simulink model "KugleSim_SlidingMode"  (R2018a)
settings: Solver=VariableStepAuto  StartTime=0.0  StopTime=5  FixedStep=1e-3  MaxStep=1e-2  RelTol=1e-5
PreLoadFcn:
  | modelDir = fileparts(get_param(bdroot, 'FileName'));
  | addpath(fullfile(modelDir,'../Parameters'));
  | addpath(fullfile(modelDir,'subsystems'));
  | 
  | Parameters_General
  | Parameters_Simulation
  | Parameters_Controllers
InitFcn:
  | Parameters_General
  | Parameters_Simulation
  | Parameters_Controllers
StopFcn:
  | StructurizeLoggedData
values from neighbouring files (symbols this model uses):
  Ts = 1/200    (= 0.005)    [Parameters_Controller.m]
settings Model: Creator=Thomas  LastModifiedBy=Thomas
settings DebuggingCC: UniqueDataStoreMsg=error
settings HardwareCC: ProdBitPerPointer=32  ProdBitPerSizeT=32  ProdBitPerPtrDiffT=32  ProdLargestAtomicInteger=Long  ProdLargestAtomicFloat=Double  ProdWordSize=32  ProdHWDeviceType=ARM Compatible->ARM Cortex
settings ModelReferenceCC: ModelReferenceNumInstancesAllowed=Zero
settings RTWCC: GenCodeOnly=on  Toolchain=GNU Tools for ARM Embedded Processors
settings GRTTargetCC: TargetLangStandard=C89/C90 (ANSI)  CodeReplacementLibrary=ARM Cortex-M (CMSIS)

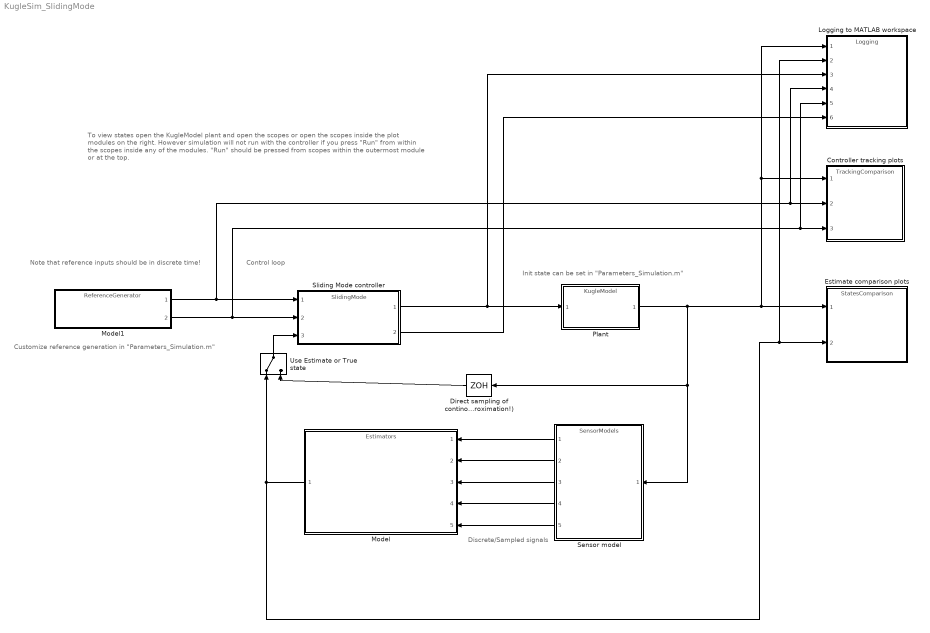
== system KugleSim_SlidingMode ==
  note: Control loop
  note: Discrete/Sampled signals
  note: Init state can be set in "Parameters_Simulation.m"
  note: To view states open the KugleModel plant and open the scopes or open the scopes inside the plot modules on the right.
      | However simulation will not run with the controller if you press "Run" from within the scopes inside any of the modules.
      | "Run" should be pressed from scopes within the outermost module or at the top.
  note: Note that reference inputs should be in discrete time!
  note: Customize reference generation in "Parameters_Simulation.m"
  Controller tracking plots : ModelReference  ModelNameDialog=TrackingComparison  SimulationMode=Normal  ModelReferenceVersion=1.12
  Direct sampling of continous states (simple/approximation!) : ZeroOrderHold  SampleTime=Ts
  Estimate comparison plots : ModelReference  ModelNameDialog=StatesComparison  SimulationMode=Normal  ModelReferenceVersion=1.9
  Logging to MATLAB workspace : ModelReference  ModelNameDialog=Logging  SimulationMode=Normal  ModelReferenceVersion=1.12
  Model : ModelReference  ModelNameDialog=Estimators  SimulationMode=Normal  ModelReferenceVersion=1.10
  Model1 : ModelReference  ModelNameDialog=ReferenceGenerator  SimulationMode=Normal  ModelReferenceVersion=1.7
  Plant : ModelReference  ModelNameDialog=KugleModel  SimulationMode=Normal  ModelReferenceVersion=1.2090
  Sensor model : ModelReference  ModelNameDialog=SensorModels  SimulationMode=Normal  ModelReferenceVersion=1.18
  Sliding Mode controller : ModelReference  ModelNameDialog=SlidingMode  SimulationMode=Normal  ModelReferenceVersion=1.48
  Use Estimate or True state : ManualSwitch
  wires:
  Direct sampling of continous states (simple/approximation!)/1 -> Use Estimate or True state/2
  Plant/1 -> Sensor model/1, Direct sampling of continous states (simple/approximation!)/1, Logging to MATLAB workspace/1, Controller tracking plots/1, Estimate comparison plots/1
  Model1/2 -> Logging to MATLAB workspace/5, Controller tracking plots/3, Sliding Mode controller/2
  Sliding Mode controller/1 -> Logging to MATLAB workspace/3, Plant/1
  Use Estimate or True state/1 -> Sliding Mode controller/3
  Sensor model/5 -> Model/5
  Sensor model/4 -> Model/4
  Sensor model/2 -> Model/2
  Sensor model/3 -> Model/3
  Sensor model/1 -> Model/1
  Model/1 -> Use Estimate or True state/1, Logging to MATLAB workspace/2, Estimate comparison plots/2
  Sliding Mode controller/2 -> Logging to MATLAB workspace/6
  Model1/1 -> Logging to MATLAB workspace/4, Controller tracking plots/2, Sliding Mode controller/1
